simulink model "fz7_4"  (R2014a)
settings: Solver=ode45  StartTime=0.0  StopTime=10.0  RelTol=1e-3
values from neighbouring files (symbols this model uses):
  SymbolRate = 1000    [eg7_11.m]    (also in eg7_2.m = 2; eg7_4.m = 2; eg7_7.m = 2)
libraries: commutil2 x4, commsink2 x2, commfilt2 x2, commdigbbndpm3 x2, commchan3 x1, commrandsrc2 x1
settings Model: Creator=tzb  LastModifiedBy=tzb
settings DebuggingCC: SolverPrmCheckMsg=none

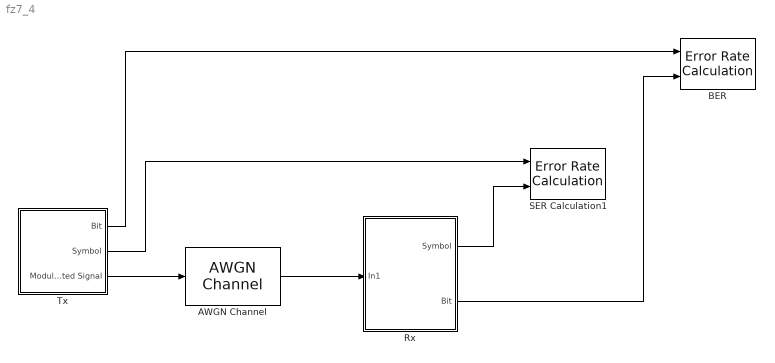
== system fz7_4 ==
  AWGN Channel : commchan3/AWGN Channel  InputProcessing=Columns as channels (frame based)  seed=67  noiseMode="Signal to noise ratio  (Es/No)"  EbNodB=10  EsNodB=SNR  SNRdB=10  bitsPerSym=1  Ps=1  Tsym=1/SymbolRate  variance=1
  BER : commsink2/Error Rate Calculation  N=0  st_delay=0  cp_mode=Entire frame  subframe=[]  PMode=Workspace  WsName=ErrorVec  RsMode2=off  stop=off  numErr=100  maxBits=1e6
  Rx : Subsystem
  SER Calculation1 : commsink2/Error Rate Calculation  N=0  st_delay=0  cp_mode=Entire frame  subframe=[]  PMode=Workspace  WsName=SER  RsMode2=off  stop=off  numErr=100  maxBits=1e6
  Tx : Subsystem
  wires:
  Tx/3(Modulated Signal) -> AWGN Channel/1
  AWGN Channel/1 -> Rx/1(In1)
  Rx/1(Symbol) -> SER Calculation1/2
  Tx/2(Symbol) -> SER Calculation1/1
  Tx/1(Bit) -> BER/1
  Rx/2(Bit) -> BER/2

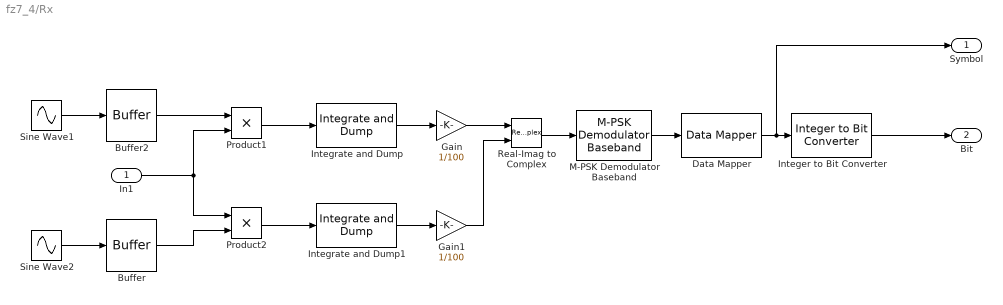
== system fz7_4/Rx ==
  In1 : Inport
  Buffer : Buffer  N=100*SymbolRate
  Buffer2 : Buffer  N=100*SymbolRate
  Data Mapper : commutil2/Data Mapper  MapMode=Gray to Binary  M=16  MapVec=[0 1 3 2 7 6 4 5]
  Gain : Gain  Gain=1/100
  Gain1 : Gain  Gain=1/100
  Integer to Bit Converter : commutil2/Integer to Bit Converter  nbits=4  signedInputValues=Unsigned  bitOrder=MSB first  outDtype=Inherit via internal rule
  Integrate and Dump : commfilt2/Integrate and Dump  obssamples=100  offsetsamples=0  nodump=off  roundingMode=Floor  overflowMode=off
  Integrate and Dump1 : commfilt2/Integrate and Dump  obssamples=100  offsetsamples=0  nodump=off  roundingMode=Floor  overflowMode=off
  M-PSK Demodulator Baseband : commdigbbndpm3/M-PSK Demodulator Baseband  M=16  Ph=0  Dec=Gray  Mapping=[0:7]  OutType=Integer  DecType=Hard decision  VarSource=Dialog  Variance=1  outDtype1=Inherit via internal rule  outDtype2=Inherit via internal rule  derotateFactorWordLen=16
  Product1 : Product
  Product2 : Product
  Real-Imag to Complex : RealImagToComplex
  Sine Wave1 : Sin  Amplitude=sqrt(2)  Frequency=2*pi*SymbolRate  Phase=pi/2  SampleTime=1/(100*SymbolRate)
  Sine Wave2 : Sin  Amplitude=sqrt(2)  Frequency=2*pi*SymbolRate  Phase=pi  SampleTime=1/(100*SymbolRate)
  Symbol : Outport
  Bit : Outport  Port=2
  wires:
  Gain/1 -> Real-Imag to Complex/1
  Integrate and Dump1/1 -> Gain1/1
  Buffer/1 -> Product2/2
  Sine Wave1/1 -> Buffer2/1
  Integer to Bit Converter/1 -> Bit/1
  Buffer2/1 -> Product1/1
  Integrate and Dump/1 -> Gain/1
  Sine Wave2/1 -> Buffer/1
  Product1/1 -> Integrate and Dump/1
  M-PSK Demodulator Baseband/1 -> Data Mapper/1
  In1/1 -> Product1/2, Product2/1
  Data Mapper/1 -> Symbol/1, Integer to Bit Converter/1
  Gain1/1 -> Real-Imag to Complex/2
  Product2/1 -> Integrate and Dump1/1
  Real-Imag to Complex/1 -> M-PSK Demodulator Baseband/1

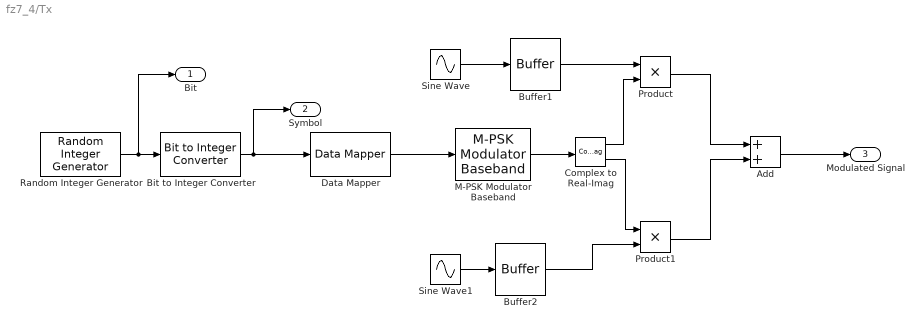
== system fz7_4/Tx ==
  Add : Sum
  Bit to Integer Converter : commutil2/Bit to Integer Converter  nbits=4  bitOrder=MSB first  signedOutputValues=Unsigned  outDtype=Inherit via internal rule  outDtypeSigned=Inherit via internal rule
  Buffer1 : Buffer  N=100*SymbolRate
  Buffer2 : Buffer  N=100*SymbolRate
  Complex to Real-Imag : ComplexToRealImag
  Data Mapper : commutil2/Data Mapper  MapMode=Binary to Gray  M=16  MapVec=[0 1 3 2 7 6 4 5]
  M-PSK Modulator Baseband : commdigbbndpm3/M-PSK Modulator Baseband  M=16  InType=Integer  Enc=Gray  Mapping=[0:7]  Ph=pi/8  outDtype=double  outWordLen=16  outUDDataType=sfix(16)  outFracLenMode=Best precision  outFracLen=15
  Product : Product
  Product1 : Product
  Random Integer Generator : commrandsrc2/Random Integer Generator  mul=2  seed=37  Ts=1/(4*SymbolRate)  frameBased=on  sampPerFrame=4*SymbolRate  orient=off  outDataType=double
  Sine Wave : Sin  Amplitude=sqrt(2)  Frequency=2*pi*SymbolRate  Phase=pi/2  SampleTime=1/(100*SymbolRate)
  Sine Wave1 : Sin  Amplitude=sqrt(2)  Frequency=2*pi*SymbolRate  Phase=pi  SampleTime=1/(100*SymbolRate)
  Bit : Outport
  Symbol : Outport  Port=2
  Modulated Signal : Outport  Port=3
  wires:
  Add/1 -> Modulated Signal/1
  Product1/1 -> Add/2
  Bit to Integer Converter/1 -> Symbol/1, Data Mapper/1
  Sine Wave/1 -> Buffer1/1
  M-PSK Modulator Baseband/1 -> Complex to Real-Imag/1
  Complex to Real-Imag/1 -> Product/2
  Complex to Real-Imag/2 -> Product1/1
  Sine Wave1/1 -> Buffer2/1
  Buffer2/1 -> Product1/2
  Product/1 -> Add/1
  Buffer1/1 -> Product/1
  Random Integer Generator/1 -> Bit/1, Bit to Integer Converter/1
  Data Mapper/1 -> M-PSK Modulator Baseband/1
